simulink model "ILC_pidDCsim"  (R2024a)
settings: Solver=ode45  StartTime=time_ILC(1)  StopTime=time_ILC(end)  RelTol=1e-3  AbsTol=1e-6
PreLoadFcn:
  | ILC_setup
values from neighbouring files (symbols this model uses):
  tsamp_ILC = 0.010    (= 0.01)    [ILC_setup.m]
libraries: slctrlobsolete x2, simulink x1
settings Model: Creator=stefan  LastModifiedBy=marmr
settings SolverCC: AutoScaleAbsTol=off  AlgebraicLoopSolver=TrustRegion
settings DataIOCC: SaveFormat=Array  SignalLoggingSaveFormat=ModelDataLogs  ReturnWorkspaceOutputs=off
settings OptimizationCC: BooleanDataType=off  ReuseModelBlockBuffer=off  ExpressionDepthLimit=2147483647  LifeSpan=inf
settings DebuggingCC: SaveWithParameterizedLinksMsg=none  UnderspecifiedInitializationDetection=Classic  MergeDetectMultiDrivingBlocksExec=none  SignalResolutionControl=TryResolveAllWithWarning  MultiTaskDSMMsg=warning  MultiTaskCondExecSysMsg=none  FcnCallInpInsideContextMsg=warning  UnconnectedInputMsg=warning  UnconnectedOutputMsg=warning  UnconnectedLineMsg=warning  StateNameClashWarn=warning  SFUnexpectedBacktrackingDiag=warning  SFNoUnconditionalDefaultTransitionDiag=warning  SFExecutionAtInitializationDiag=none  ArithmeticOperatorsInVariantConditions=warning
settings HardwareCC: ProdBitPerPointer=32  ProdBitPerSizeT=32  ProdBitPerPtrDiffT=32  ProdLargestAtomicFloat=None  ProdIntDivRoundTo=Undefined  ProdEndianess=Unspecified  ProdWordSize=32  ProdHWDeviceType=32-bit Generic  TargetUnknown=on
settings ModelReferenceCC: EnableRefExpFcnMdlSchedulingChecks=on  PropagateSignalLabelsOutOfModel=off
settings SFSimCC: SimUseLocalCustomCode=off  CustomCodeUndefinedFunction=UseInterfaceOnly
settings RTWCC: RTWUseLocalCustomCode=off  GPUComputeCapability=3.5  DLArmComputeVersion=19.05
settings CodeAppCC: StateflowObjectComments=on
settings GRTTargetCC: TargetLangStandard=C89/C90 (ANSI)  CombineOutputUpdateFcns=off  GRTInterface=on
settings ConfigComp: CovMetricSettings=dw  CovSaveCumulativeToWorkspaceVar=on  CovSaveSingleToWorkspaceVar=on  CovExternalEMLEnable=off

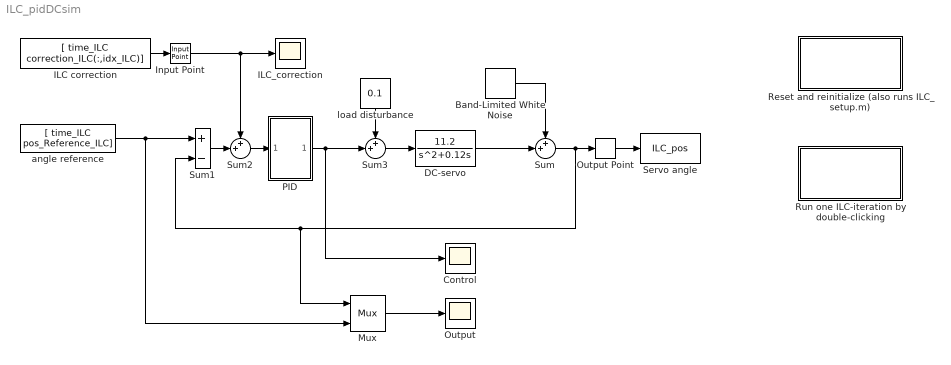
== system ILC_pidDCsim ==
  Band-Limited White Noise : simulink/Sources/Band-Limited White Noise  Cov=[0.0001]*0  Ts=0.1  seed=[23341]
  Control : Scope
  DC-servo : TransferFcn  Numerator=[11.2]  Denominator=[1 0.12 0]
  ILC correction : FromWorkspace  VariableName=[ time_ILC correction_ILC(:,idx_ILC)]  SampleTime=tsamp_ILC  ZeroCross=off
  ILC_correction : Scope
  Input Point : slctrlobsolete/Input Point
  Mux : Mux  Inputs=2
  Output : Scope
  Output Point : slctrlobsolete/Output Point
  PID : Subsystem  mask{K=1, Ti=10, Td=0.5}
  Reset and reinitialize (also runs ILC_setup.m) : Subsystem
      settings: OpenFcn=reset_idx_ILC
      mask Display: disp(['Reset-ILC (=' evalin('base','num2str(idx_ILC)') ')' ])
  Run one ILC-iteration by double-clicking : Subsystem
      settings: OpenFcn=run_ILC_iteration
      mask Display:
      | %disp(['ILC-iteration (' num2str(idx_ILC) ')' ])
      | disp(['ILC-iteration (=' evalin('base','num2str(idx_ILC)') ')' ])
  Servo angle : ToWorkspace  VariableName=ILC_pos  SaveFormat=Structure With Time  SampleTime=-1
  Sum : Sum  Inputs=++|  InputSameDT=on  SaturateOnIntegerOverflow=on  OutDataTypeStr=Inherit: Same as first input
  Sum1 : Sum  Inputs=+-  InputSameDT=on  SaturateOnIntegerOverflow=on  OutDataTypeStr=Inherit: Same as first input
  Sum2 : Sum  Inputs=++|  InputSameDT=on  SaturateOnIntegerOverflow=on  OutDataTypeStr=Inherit: Same as first input
  Sum3 : Sum  Inputs=++|  InputSameDT=on  SaturateOnIntegerOverflow=on  OutDataTypeStr=Inherit: Same as first input
  angle reference : FromWorkspace  VariableName=[ time_ILC pos_Reference_ILC]  SampleTime=tsamp_ILC  ZeroCross=off
  load disturbance : Constant  Value=0.1
  wires:
  Mux/1 -> Output/1
  PID/1(Out1) -> Control/1, Sum3/2
  DC-servo/1 -> Sum/2
  Sum/1 -> Mux/1, Sum1/2, Output Point/1
  Band-Limited White Noise/1 -> Sum/1
  Output Point/1 -> Servo angle/1
  Sum2/1 -> PID/1(In1)
  Sum1/1 -> Sum2/2
  Sum3/1 -> DC-servo/1
  angle reference/1 -> Mux/2, Sum1/1
  load disturbance/1 -> Sum3/1
  ILC correction/1 -> Input Point/1
  Input Point/1 -> ILC_correction/1, Sum2/1

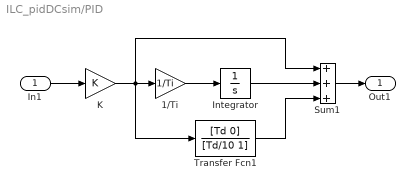
== system ILC_pidDCsim/PID ==
  In1 : Inport
  1/Ti : Gain  Gain=1/Ti  SaturateOnIntegerOverflow=on  OutDataTypeStr=Inherit: Same as input  ParamDataTypeStr=Inherit: Same as input
  Integrator : Integrator
  K : Gain  Gain=K  SaturateOnIntegerOverflow=on  OutDataTypeStr=Inherit: Same as input  ParamDataTypeStr=Inherit: Same as input
  Sum1 : Sum  Inputs=+++  InputSameDT=on  SaturateOnIntegerOverflow=on  OutDataTypeStr=Inherit: Same as first input
  Transfer Fcn1 : TransferFcn  Numerator=[Td 0]  Denominator=[Td/10 1]
  Out1 : Outport
  wires:
  In1/1 -> K/1
  K/1 -> 1/Ti/1, Transfer Fcn1/1, Sum1/1
  1/Ti/1 -> Integrator/1
  Sum1/1 -> Out1/1
  Integrator/1 -> Sum1/2
  Transfer Fcn1/1 -> Sum1/3

== system ILC_pidDCsim/Reset and reinitialize (also runs ILC_setup.m) ==

== system ILC_pidDCsim/Run one ILC-iteration by double-clicking ==
